simulink model "longitudinal_modelV2"  (R2023a)
settings: Solver=VariableStepAuto  StartTime=0.0  StopTime=1100  RelTol=1e-3
undefined symbols (not defined in the file): A_f, brakeTime, breakStrength, C_alpha, C_d, C_rr, C_s, eta_t, g, headWind, headWindTime, I_w, l_f, l_r, lambda_f, lambda_t, M, Meq, motorDecrease, motorDecreaseTime, motorIncrease, motorIncreaseTime, motorStart, motorStartTime, mu, R_w, rho, roadSlopeTime
libraries: simulink x1
settings Model: Creator=Samsung  LastModifiedBy=brianlesko
settings SolverCC: AlgebraicLoopSolver=TrustRegion
settings DataIOCC: ReturnWorkspaceOutputs=off
settings OptimizationCC: ReuseModelBlockBuffer=off
settings DebuggingCC: UnconnectedInputMsg=warning  UnconnectedOutputMsg=warning  UnconnectedLineMsg=warning  ArithmeticOperatorsInVariantConditions=warning
settings ModelReferenceCC: EnableRefExpFcnMdlSchedulingChecks=on
settings SFSimCC: SimUseLocalCustomCode=off  CustomCodeUndefinedFunction=UseInterfaceOnly
settings RTWCC: RTWUseLocalCustomCode=off
settings CodeAppCC: StateflowObjectComments=on

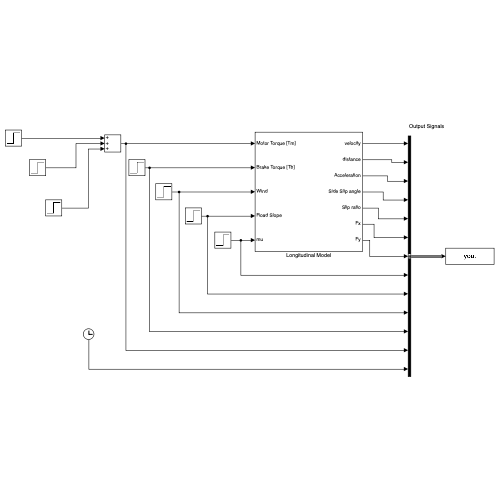
[thumbnail: Simulink's stored preview of the top-level diagram]
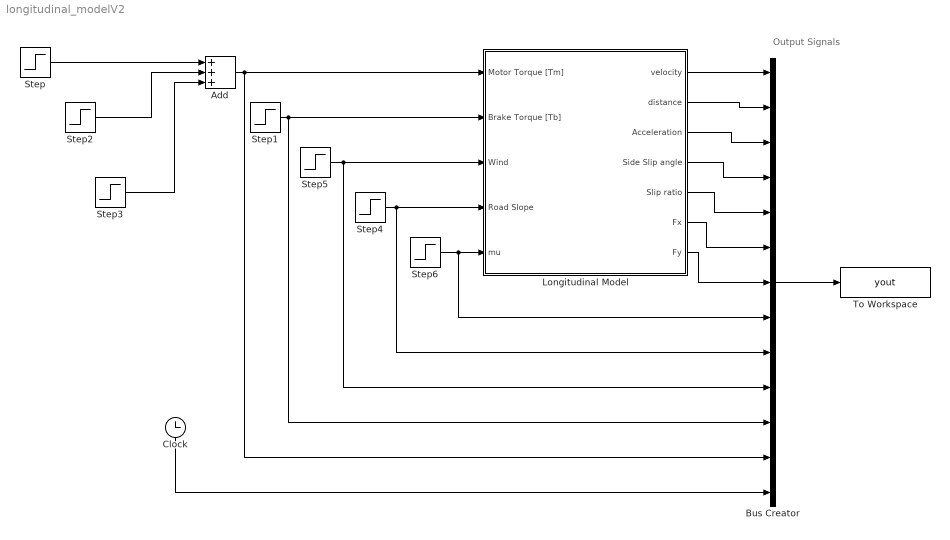
== system longitudinal_modelV2 ==
  note: Output Signals
  Add : Sum  Inputs=+++
  Bus Creator : BusCreator  Inputs=13
  Clock : Clock
  Longitudinal Model : Subsystem
  Step : Step  Time=motorStartTime  After=motorStart  SampleTime=0
  Step1 : Step  Time=brakeTime  After=breakStrength  SampleTime=0
  Step2 : Step  Time=motorIncreaseTime  After=motorIncrease  SampleTime=0
  Step3 : Step  Time=motorDecreaseTime  After=-motorDecrease  SampleTime=0
  Step4 : Step  Time=roadSlopeTime  After=roadSlopeTime  SampleTime=0
  Step5 : Step  Time=headWindTime  After=headWind  SampleTime=0
  Step6 : Step  Time=0  Before=mu  After=mu  SampleTime=0
  To Workspace : ToWorkspace  VariableName=yout  SampleTime=-1
  wires:
  Step1/1 -> Longitudinal Model/2(Brake Torque [Tb]), Bus Creator/11
  Add/1 -> Longitudinal Model/1(Motor Torque [Tm]), Bus Creator/12
  Step2/1 -> Add/2
  Step3/1 -> Add/3
  Step/1 -> Add/1
  Step5/1 -> Bus Creator/10, Longitudinal Model/3(Wind)
  Step4/1 -> Bus Creator/9, Longitudinal Model/4(Road Slope)
  Step6/1 -> Bus Creator/8, Longitudinal Model/5(mu)
  Bus Creator/1 -> To Workspace/1
  Clock/1 -> Bus Creator/13
  Longitudinal Model/7(Fy) -> Bus Creator/7
  Longitudinal Model/6(Fx) -> Bus Creator/6
  Longitudinal Model/5(Slip ratio) -> Bus Creator/5
  Longitudinal Model/4(Side Slip angle) -> Bus Creator/4
  Longitudinal Model/3(Acceleration) -> Bus Creator/3
  Longitudinal Model/2(distance) -> Bus Creator/2
  Longitudinal Model/1(velocity) -> Bus Creator/1

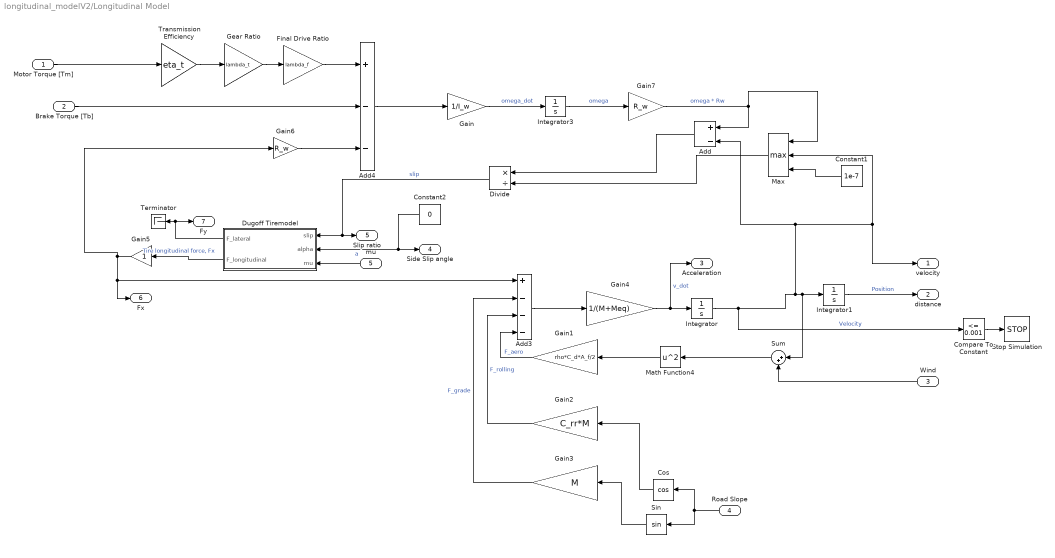
== system longitudinal_modelV2/Longitudinal Model ==
  Motor Torque [Tm] : Inport
  Brake Torque [Tb] : Inport  Port=2
  Wind : Inport  Port=3
  Road Slope : Inport  Port=4
  mu : Inport  Port=5
  Add : Sum  Inputs=+-
  Add3 : Sum  Inputs=+---
  Add4 : Sum  Inputs=+--
  Compare To Constant : simulink/Logic and Bit Operations/Compare To Constant  relop=<=  const=0.001  OutDataTypeStr=boolean
  Constant1 : Constant  Value=1e-7
  Constant2 : Constant  Value=0
  Cos : Trigonometry  Operator=cos
  Divide : Product  Inputs=*/
  Dugoff Tiremodel : Subsystem
  Final Drive Ratio : Gain  Gain=lambda_f
  Gain : Gain  Gain=1/I_w
  Gain1 : Gain  Gain=rho*C_d*A_f/2
  Gain2 : Gain  Gain=C_rr*M
  Gain3 : Gain  Gain=M
  Gain4 : Gain  Gain=1/(M+Meq)
  Gain5 : Gain
  Gain6 : Gain  Gain=R_w
  Gain7 : Gain  Gain=R_w
  Gear Ratio : Gain  Gain=lambda_t
  Integrator : Integrator  InitialCondition=0.01  LimitOutput=on  LowerSaturationLimit=0
  Integrator1 : Integrator
  Integrator3 : Integrator  InitialCondition=1
  Math Function4 : Math  Operator=square  SignedPower=on
  Max : MinMax  Function=max  Inputs=3
  Sin : Trigonometry
  Stop Simulation : Stop
  Sum : Sum  Inputs=|++
  Terminator : Terminator
  Transmission Efficiency : Gain  Gain=eta_t
  velocity : Outport  VectorParamsAs1DForOutWhenUnconnected=off
  distance : Outport  Port=2  VectorParamsAs1DForOutWhenUnconnected=off
  Acceleration : Outport  Port=3  VectorParamsAs1DForOutWhenUnconnected=off
  Side Slip angle : Outport  Port=4
  Slip ratio : Outport  Port=5
  Fx : Outport  Port=6
  Fy : Outport  Port=7
  wires:
  Integrator/1 -> Compare To Constant/1, Sum/1, Integrator1/1, velocity/1, Max/2, Add/2  "Velocity"
  Brake Torque [Tb]/1 -> Add4/2
  Compare To Constant/1 -> Stop Simulation/1
  Road Slope/1 -> Sin/1, Cos/1
  Sin/1 -> Gain3/1
  Gain2/1 -> Add3/3  "F_rolling"
  Add3/1 -> Gain4/1
  Constant2/1 -> Side Slip angle/1, Dugoff Tiremodel/2(alpha)  "a"
  Gain5/1 -> Gain6/1, Fx/1, Add3/1
  Wind/1 -> Sum/2
  Motor Torque [Tm]/1 -> Transmission Efficiency/1
  Gain7/1 -> Max/1, Add/1  "omega * Rw"
  Cos/1 -> Gain2/1
  Integrator1/1 -> distance/1  "Position"
  Gear Ratio/1 -> Final Drive Ratio/1
  Constant1/1 -> Max/3
  Gain/1 -> Integrator3/1  "omega_dot"
  Divide/1 -> Slip ratio/1, Dugoff Tiremodel/1(slip)  "slip"
  Max/1 -> Divide/2
  Final Drive Ratio/1 -> Add4/1
  Gain4/1 -> Acceleration/1, Integrator/1  "v_dot"
  Math Function4/1 -> Gain1/1
  Transmission Efficiency/1 -> Gear Ratio/1
  Integrator3/1 -> Gain7/1  "omega"
  Gain1/1 -> Add3/4  "F_aero"
  Dugoff Tiremodel/1(F_lateral) -> Terminator/1, Fy/1
  Add4/1 -> Gain/1
  Add/1 -> Divide/1
  Gain3/1 -> Add3/2  "F_grade"
  Gain6/1 -> Add4/3
  Dugoff Tiremodel/2(F_longitudinal) -> Gain5/1  "Tire longitudinal force, Fx"
  Sum/1 -> Math Function4/1
  mu/1 -> Dugoff Tiremodel/3(mu)

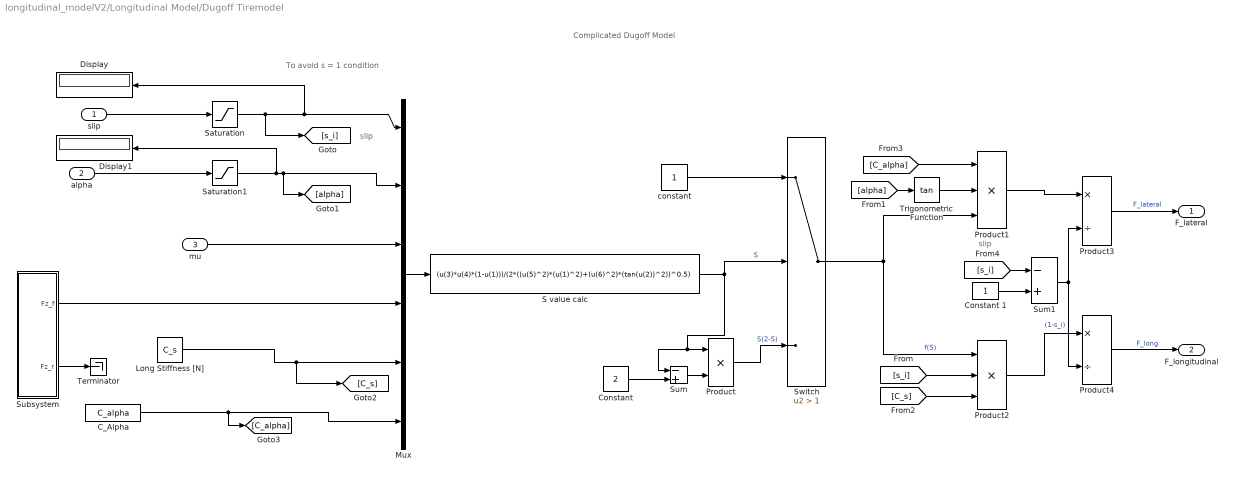
== system longitudinal_modelV2/Longitudinal Model/Dugoff Tiremodel ==
  note: slip
  note: To avoid s = 1 condition
  note: Complicated Dugoff Model
  note: slip
  slip : Inport
  alpha : Inport  Port=2
  mu : Inport  Port=3
  C_Alpha : Constant  Value=C_alpha
  "Constant " : Constant  Value=2
  Constant 1 : Constant
  Display : Display
  Display1 : Display
  Long Stiffness [N] : Constant  Value=C_s
  Mux : Mux  Inputs=6
  Product : Product
  Product1 : Product  Inputs=3
  Product2 : Product  Inputs=3
  Product3 : Product  Inputs=*/
  Product4 : Product  Inputs=*/
  S value calc : Fcn  Expr=(u(3)*u(4)*(1-u(1)))/(2*((u(5)^2)*(u(1)^2)+(u(6)^2)*(tan(u(2))^2))^0.5)
  Saturation : Saturate  UpperLimit=0.999  LowerLimit=-1
  Saturation1 : Saturate  UpperLimit=20  LowerLimit=1e-4
  Subsystem : Subsystem
  Sum : Sum  Inputs=-+
  Sum1 : Sum  Inputs=-+
  Switch : Switch  Criteria=u2 > Threshold  Threshold=1  SaturateOnIntegerOverflow=off  InputSameDT=off
  Terminator : Terminator
  Trigonometric Function : Trigonometry  Operator=tan
  constant : Constant
  F_lateral : Outport  VectorParamsAs1DForOutWhenUnconnected=off
  F_longitudinal : Outport  Port=2  VectorParamsAs1DForOutWhenUnconnected=off
  wires:
  Switch/1 -> Product2/1, Product1/3  "f(S)"
  [s_i] -> Sum1/1
  Trigonometric Function/1 -> Product1/2
  Sum1/1 -> Product3/2, Product4/2  "(1-s_i)"
  [alpha] -> Trigonometric Function/1
  [C_alpha] -> Product1/1
  [s_i] -> Product2/2
  [C_s] -> Product2/3
  Product2/1 -> Product4/1
  Product1/1 -> Product3/1
  Product4/1 -> F_longitudinal/1  "F_long"
  Constant 1/1 -> Sum1/2
  Product3/1 -> F_lateral/1  "F_lateral"
  Sum/1 -> Product/2
  Subsystem/1(Fz_f) -> Mux/4
  "Constant "/1 -> Sum/2
  Saturation/1 -> Display/1, Mux/1, [s_i]
  mu/1 -> Mux/3
  Mux/1 -> S value calc/1
  Long Stiffness [N]/1 -> [C_s], Mux/5
  S value calc/1 -> Switch/2, Product/1, Sum/1  "S"
  slip/1 -> Saturation/1
  alpha/1 -> Saturation1/1
  C_Alpha/1 -> [C_alpha], Mux/6
  Saturation1/1 -> Display1/1, [alpha], Mux/2
  constant/1 -> Switch/1
  Product/1 -> Switch/3  "S(2-S)"
  Subsystem/2(Fz_r) -> Terminator/1

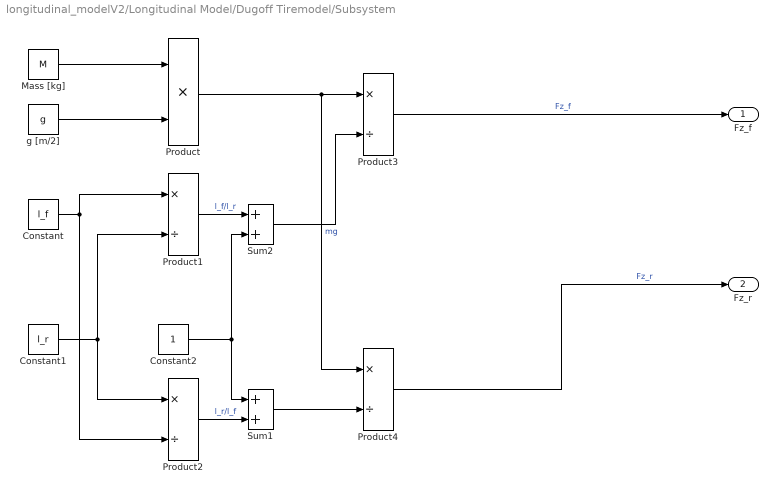
== system longitudinal_modelV2/Longitudinal Model/Dugoff Tiremodel/Subsystem ==
  Constant : Constant  Value=l_f
  Constant1 : Constant  Value=l_r
  Constant2 : Constant
  Mass [kg] : Constant  Value=M
  Product : Product  Inputs=**
  Product{1..4} (4 alike) : Product  Inputs=*/
  Sum1 : Sum
  Sum2 : Sum
  g [m/2] : Constant  Value=g
  Fz_f : Outport  VectorParamsAs1DForOutWhenUnconnected=off
  Fz_r : Outport  Port=2  VectorParamsAs1DForOutWhenUnconnected=off
  wires:
  Sum2/1 -> Product3/2
  Product2/1 -> Sum1/2  "l_r/l_f"
  Sum1/1 -> Product4/2
  Product4/1 -> Fz_r/1  "Fz_r"
  Constant1/1 -> Product2/1, Product1/2
  Product/1 -> Product3/1, Product4/1  "mg"
  Constant/1 -> Product1/1, Product2/2
  Constant2/1 -> Sum1/1, Sum2/2
  Product1/1 -> Sum2/1  "l_f/l_r"
  Product3/1 -> Fz_f/1  "Fz_f"
  Mass [kg]/1 -> Product/1
  g [m/2]/1 -> Product/2
